simulink model "PhaseShiftedCarriers"  (R2023b)
settings: Solver=FixedStepAuto  StartTime=0.0  StopTime=4/ffund  FixedStep=1e-6  RelTol=1e-3
InitFcn:
  | fsw=50e3;
  | 
  | ma=0.9;
  | 
  | ffund=100;
  | 
  | phi_pf=acos(0.9);
  | % 15*pi/180;
  | 
  | sym= pi/6;
libraries: spsRMSLib x5, dspstat3 x2, simulink x1
settings Model: Creator=enesa  LastModifiedBy=enesa

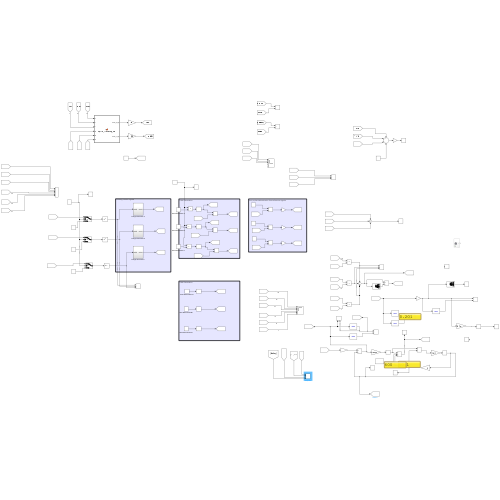
[thumbnail: Simulink's stored preview of the top-level diagram]
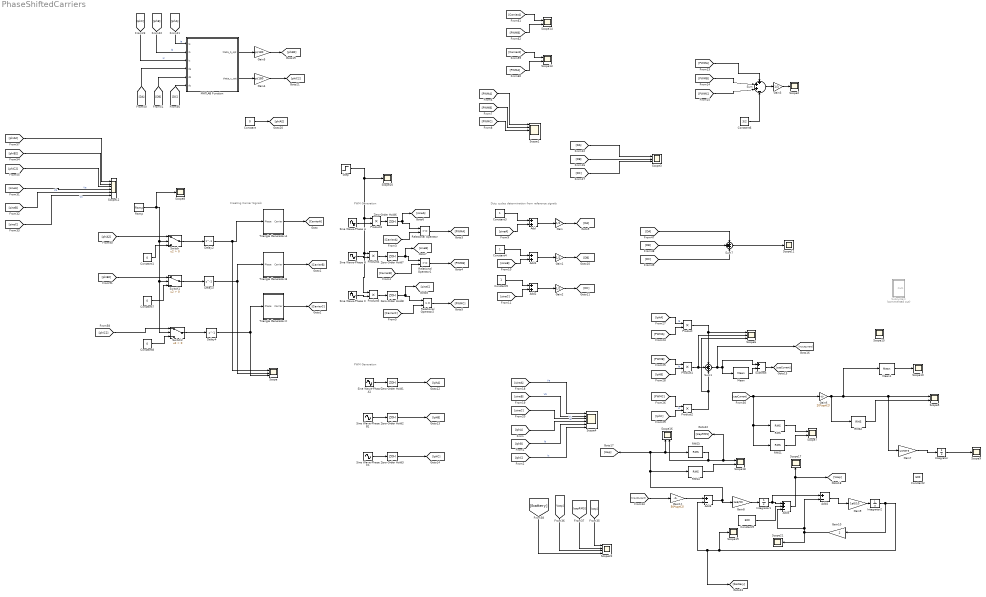
== system PhaseShiftedCarriers ==
  note: Duty cycles determination from reference signals
  note: PWM Generation
  note: Creating Carrier Signals
  note: PWM Generation
  Add : Sum
  Add1 : Sum
  Add2 : Sum
  Add3 : Sum  Inputs=+-
  Add4 : Sum  Inputs=+-
  Add5 : Sum  Inputs=++-
  Constant{,1,7..8} (4 alike) : Constant  Value=0
  Constant2 : Constant  Value=600
  Constant3 : Constant
  Constant4 : Constant
  Constant5 : Constant
  Constant6 : Constant  Value=3/2
  Constant9 : Constant  Value=600
  Delay2 : Delay  DelayLength=1  SampleTime=1/fsw
  Delay3 : Delay  DelayLength=1  SampleTime=1/fsw
  Delay4 : Delay  DelayLength=1  SampleTime=1/fsw
  Gain : Gain  Gain=1/2
  Gain1 : Gain  Gain=1/2
  Gain10 : Gain  Gain=2
  Gain11 : Gain  Gain=50*sqrt(2)
  Gain2 : Gain  Gain=1/2
  Gain3 : Gain  Gain=1/3
  Gain4 : Gain  Gain=pi/180
  Gain5 : Gain  Gain=pi/180
  Gain6 : Gain  Gain=20*sqrt(2)
  Gain7 : Gain  Gain=1/470e-6
  Gain8 : Gain  Gain=1e6/50
  Gain9 : Gain  Gain=1e6/10
  Integrator : Integrator
  Integrator1 : Integrator
  Integrator2 : Integrator
  MATLAB Function : MATLAB Function  TreatAsAtomicUnit=on
  Mean : dspstat3/Mean  run=on  InputProcessing=Columns as channels (frame based)  reset_popup=None  directionMode=Each column  dimension=1  roiEnable=off  roiType=Rectangles  roiPortion=Entire ROI  roiOutput=Individual statistics for each ROI  roiFlag=off  roundingMode=Floor  overflowMode=off  outputDataTypeStr=Inherit: Same as accumulator  outputMin=[]  outputMax=[]  outputLastDataTypeStr=Inherit: Same as accumulator
  Mean1 : dspstat3/Mean  run=on  reset_popup=None  directionMode=Each column  dimension=1  roiEnable=off  roiType=Rectangles  roiPortion=Entire ROI  roiOutput=Individual statistics for each ROI  roiFlag=off  roundingMode=Floor  overflowMode=off  outputDataTypeStr=Inherit: Same as accumulator  outputMin=[]  outputMax=[]  outputLastDataTypeStr=Inherit: Same as accumulator
  Product{,1..5} (6 alike) : Product
  RMS : spsRMSLib/RMS  TrueRMS=on  Freq=fsw  RMSInit=0  Ts=0
  RMS1 : spsRMSLib/RMS  TrueRMS=on  Freq=ffund  RMSInit=0  Ts=0
  RMS2 : spsRMSLib/RMS  TrueRMS=on  Freq=fsw  RMSInit=0  Ts=0
  RMS3 : spsRMSLib/RMS  TrueRMS=on  Freq=fsw  RMSInit=0  Ts=0
  RMS4 : spsRMSLib/RMS  TrueRMS=on  Freq=ffund  RMSInit=0  Ts=0
  Ramp : simulink/Sources/Ramp  slope=ffund/2  start=0  InitialOutput=-1
  Relational Operator : RelationalOperator  OutDataTypeStr=boolean  RndMeth=Simplest  InputSameDT=off
  Relational Operator1 : RelationalOperator  OutDataTypeStr=boolean  RndMeth=Simplest  InputSameDT=off
  Relational Operator2 : RelationalOperator  OutDataTypeStr=boolean  RndMeth=Simplest  InputSameDT=off
  Scope : Scope  NumInputPorts=3
  Scope1 : Scope  NumInputPorts=6
  Scope{2,8..11,15,17,19..21} (10 alike) : Scope
  Scope12 : Scope  NumInputPorts=6
  Scope{5,7,13..14,16,18} (6 alike) : Scope  NumInputPorts=2
  Scope22 : Scope  NumInputPorts=4
  Scope3 : Scope  NumInputPorts=3
  Scope4 : Scope  NumInputPorts=6
  Scope6 : Scope  NumInputPorts=3
  Sine Wave-Phase A : Sin  Amplitude=ma  Frequency=2*pi*ffund  SampleTime=0
  Sine Wave-Phase A1 : Sin  Amplitude=ma  Frequency=2*pi*ffund  Phase=0-phi_pf  SampleTime=0
  Sine Wave-Phase B : Sin  Amplitude=ma  Frequency=2*pi*ffund  Phase=2*pi/3  SampleTime=0
  Sine Wave-Phase B1 : Sin  Amplitude=ma  Frequency=2*pi*ffund  Phase=2*pi/3-phi_pf  SampleTime=0
  Sine Wave-Phase C : Sin  Amplitude=ma  Frequency=2*pi*ffund  Phase=-2*pi/3  SampleTime=0
  Sine Wave-Phase C1 : Sin  Amplitude=ma  Frequency=2*pi*ffund  Phase=-2*pi/3-phi_pf  SampleTime=0
  Step : Step  Time=8/ffund  Before=0.6/0.9  SampleTime=0
  Subsystem : Subsystem  Commented=on
  Subtract : Sum  Inputs=+-
  Sum : Sum  Inputs=+++-
  Sum1 : Sum  Inputs=+++
  Sum7 : Sum  Inputs=+++
  Switch : Switch  Criteria=u2 > Threshold  SaturateOnIntegerOverflow=off  InputSameDT=off
  Switch1 : Switch  Criteria=u2 > Threshold  SaturateOnIntegerOverflow=off  InputSameDT=off
  Switch2 : Switch  Criteria=u2 > Threshold  SaturateOnIntegerOverflow=off  InputSameDT=off
  Triangle Generator-A : Subsystem
  Triangle Generator-B : Subsystem
  Triangle Generator-C : Subsystem
  Zero-Order Hold{1..3,6..8} (6 alike) : ZeroOrderHold  SampleTime=5/fsw
  wires:
  [PWMA] -> Scope1/1
  [PWMB] -> Scope1/2
  [PWMC] -> Scope1/3
  [PWMA] -> Sum/1
  [PWMB] -> Sum/2
  [PWMC] -> Sum/3
  Sum/1 -> Gain3/1
  Gain3/1 -> Scope2/1
  Constant6/1 -> Sum/4
  [DA] -> Scope3/1
  [DB] -> Scope3/2
  [DC] -> Scope3/3
  Triangle Generator-C/1(Carrier) -> [CarrierC]
  Triangle Generator-B/1(Carrier) -> [CarrierB]
  Triangle Generator-A/1(Carrier) -> [CarrierA]
  [CarrierB] -> Relational Operator1/2
  Relational Operator1/1 -> [PWMB]
  Relational Operator/1 -> [PWMA]
  Relational Operator2/1 -> [PWMC]
  [CarrierC] -> Relational Operator2/2
  [CarrierA] -> Relational Operator/2
  [sineC] -> Add2/2
  Constant4/1 -> Add1/1
  Constant3/1 -> Add/1
  Add2/1 -> Gain2/1
  Gain/1 -> [DA]
  Gain2/1 -> [DC]
  Add1/1 -> Gain1/1
  [sineB] -> Add1/2
  Constant5/1 -> Add2/1
  [sineA] -> Add/2
  Gain1/1 -> [DB]
  Add/1 -> Gain/1
  [DA] -> Sum7/1
  [DC] -> Sum7/3
  [DB] -> Sum7/2
  Sum7/1 -> Scope11/1
  [phiB2] -> Scope12/2
  [phiC2] -> Scope12/3
  [phiA2] -> Scope12/1
  [CarrierA] -> Scope13/1
  [PWMA] -> Scope13/2
  [CarrierA] -> Scope14/1
  [PWMB] -> Scope14/2
  Gain4/1 -> [phiC2]
  Constant/1 -> [phiA2]
  Zero-Order Hold6/1 -> Relational Operator/1, [sineA]
  Zero-Order Hold7/1 -> [sineB], Relational Operator1/1
  Zero-Order Hold8/1 -> Relational Operator2/1, [sineC]
  Delay2/1 -> Scope/1, Triangle Generator-A/1(Phase)
  Delay3/1 -> Triangle Generator-B/1(Phase), Scope/2
  Delay4/1 -> Triangle Generator-C/1(Phase), Scope/3
  Zero-Order Hold1/1 -> [IphA]
  Zero-Order Hold2/1 -> [IphB]
  Sine Wave-Phase C1/1 -> Zero-Order Hold3/1
  Sine Wave-Phase B1/1 -> Zero-Order Hold2/1
  Zero-Order Hold3/1 -> [IphC]
  Sine Wave-Phase A1/1 -> Zero-Order Hold1/1
  [sineA] -> Scope4/1  "Va"
  [sineB] -> Scope4/2  "Vb"
  [sineC] -> Scope4/3  "Vc"
  [IphA] -> Scope4/4  "Ia"
  [IphB] -> Scope4/5  "Ib"
  [IphC] -> Scope4/6  "Ic"
  [DA] -> MATLAB Function/4(da)
  [DB] -> MATLAB Function/5(db)
  [DC] -> MATLAB Function/6(dc)
  [IphA] -> MATLAB Function/1(ia)  "Ia"
  [IphB] -> MATLAB Function/2(ib)  "Ib"
  [IphC] -> MATLAB Function/3(ic)  "Ic"
  MATLAB Function/1(theta_b_opt) -> Gain5/1
  MATLAB Function/2(theta_c_opt) -> Gain4/1
  Gain5/1 -> [phiB2]
  [IphA] -> Product/1  "Ia"
  [PWMA] -> Product/2
  [PWMB] -> Product1/1
  [IphB] -> Product1/2  "Ib"
  [PWMC] -> Product2/1
  [IphC] -> Product2/2  "Ic"
  Product/1 -> Sum1/1, Scope6/1
  Product1/1 -> Scope6/2, Sum1/2
  Product2/1 -> Scope6/3, Sum1/3
  [capCurrent] -> RMS1/1, RMS/1, Gain6/1
  Switch/1 -> Delay2/1
  [phiA2] -> Switch/1
  Constant1/1 -> Switch/3
  Ramp/1 -> Scope8/1, Switch2/2, Switch1/2, Switch/2
  Switch1/1 -> Delay3/1
  Constant7/1 -> Switch1/3
  [phiB2] -> Switch1/1
  Switch2/1 -> Delay4/1
  [phiC2] -> Switch2/1
  Constant8/1 -> Switch2/3
  RMS/1 -> Scope7/1
  [sineA] -> Scope12/4  "Va"
  [sineB] -> Scope12/5  "Vb"
  [sineC] -> Scope12/6  "Vc"
  RMS1/1 -> Scope7/2
  Sum1/1 -> [InputCurrent], Mean/1, Subtract/1
  Mean/1 -> Subtract/2
  Subtract/1 -> [capCurrent]
  Gain6/1 -> RMS2/1, Mean1/1, Gain7/1, Scope5/1
  RMS2/1 -> Scope5/2
  Gain7/1 -> Integrator/1
  Integrator/1 -> Scope9/1
  Mean1/1 -> Scope10/1
  [InputCurrent] -> Gain11/1
  Gain8/1 -> Integrator1/1
  Add4/1 -> Gain9/1
  Gain9/1 -> Integrator2/1
  Integrator2/1 -> Scope19/1, [Ibattery], Add3/2, Gain10/1
  Gain10/1 -> Add5/3, Add4/2, Scope21/1
  Integrator1/1 -> Add4/1, Add5/1
  Add5/1 -> Scope17/1, [Vcap]
  Gain11/1 -> Add3/1
  RMS4/1 -> Scope18/2
  Add3/1 -> Gain8/1, RMS3/1, Scope16/1, [Icap], RMS4/1
  RMS3/1 -> Scope16/2, [IcapRMS], Scope18/1
  Product3/1 -> Zero-Order Hold6/1
  Sine Wave-Phase A/1 -> Product3/2
  Step/1 -> Scope20/1, Product3/1, Product5/1, Product4/1
  Product4/1 -> Zero-Order Hold7/1
  Sine Wave-Phase B/1 -> Product4/2
  Product5/1 -> Zero-Order Hold8/1
  Sine Wave-Phase C/1 -> Product5/2
  Constant9/1 -> Add5/2
  [Icap] -> Scope22/1
  [Vcap] -> Scope22/3
  [IcapRMS] -> Scope22/2
  [Ibattery] -> Scope22/4

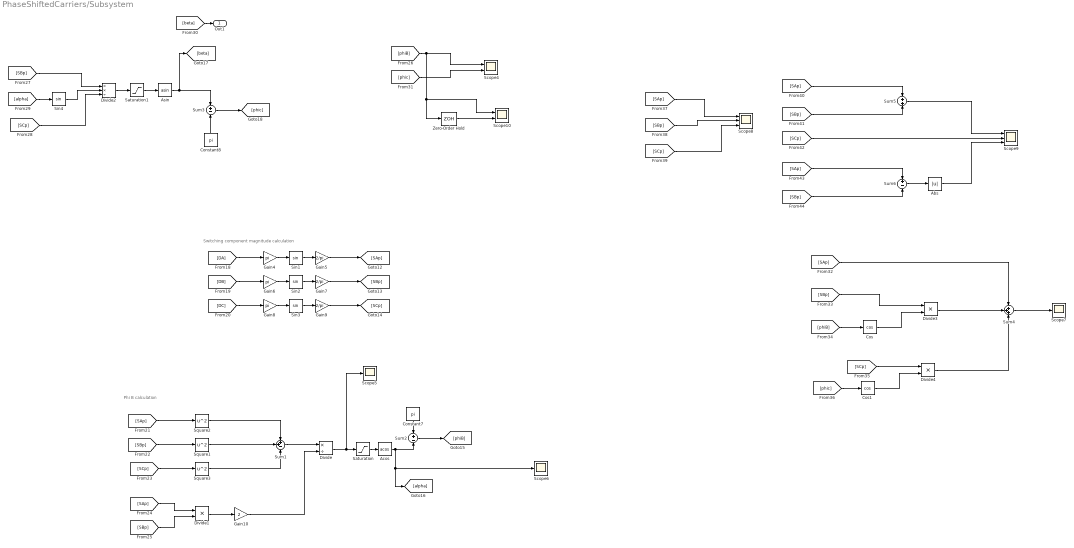
== system PhaseShiftedCarriers/Subsystem ==
  note: Phi B calculation
  note: Switching component magnitude calculation
  Abs : Abs  SaturateOnIntegerOverflow=off
  Acos : Trigonometry  Operator=acos
  Asin : Trigonometry  Operator=asin
  Constant7 : Constant  Value=pi
  Constant8 : Constant  Value=pi
  Cos : Trigonometry  Operator=cos
  Cos1 : Trigonometry  Operator=cos
  Divide : Product  Inputs=*/
  Divide1 : Product  Inputs=**
  Divide2 : Product  Inputs=**/
  Divide3 : Product  Inputs=**
  Divide4 : Product  Inputs=**
  Gain10 : Gain  Gain=2
  Gain4 : Gain  Gain=pi
  Gain5 : Gain  Gain=2/pi
  Gain6 : Gain  Gain=pi
  Gain7 : Gain  Gain=2/pi
  Gain8 : Gain  Gain=pi
  Gain9 : Gain  Gain=2/pi
  Saturation : Saturate  UpperLimit=1  LowerLimit=-1
  Saturation1 : Saturate  UpperLimit=1  LowerLimit=-1
  Scope10 : Scope  NumInputPorts=2
  Scope4 : Scope  NumInputPorts=2
  Scope5 : Scope
  Scope6 : Scope
  Scope7 : Scope
  Scope8 : Scope  NumInputPorts=3
  Scope9 : Scope  NumInputPorts=3
  Sin{1..4} (4 alike) : Trigonometry
  Square1 : Math  Operator=square
  Square2 : Math  Operator=square
  Square3 : Math  Operator=square
  Sum1 : Sum  Inputs=++-
  Sum2 : Sum  Inputs=+-
  Sum3 : Sum  Inputs=+-
  Sum4 : Sum  Inputs=+++
  Sum5 : Sum
  Sum6 : Sum  Inputs=+-
  Zero-Order Hold : ZeroOrderHold  SampleTime=1/fsw
  Out1 : Outport
  wires:
  Gain7/1 -> [SBp]
  Gain4/1 -> Sin1/1
  [SBp] -> Divide1/2
  Gain9/1 -> [SCp]
  Acos/1 -> Sum2/2, Scope6/1, [alpha]
  [beta] -> Out1/1
  Divide1/1 -> Gain10/1
  Asin/1 -> Sum3/1, [beta]
  Sin4/1 -> Divide2/2
  Gain6/1 -> Sin2/1
  Sin2/1 -> Gain7/1
  [DA] -> Gain4/1
  Gain10/1 -> Divide/2
  Gain5/1 -> [SAp]
  Sum1/1 -> Divide/1
  Square3/1 -> Sum1/3
  Square2/1 -> Sum1/1
  [SAp] -> Divide1/1
  [SBp] -> Square1/1
  Sum2/1 -> [phiB]
  [alpha] -> Sin4/1
  [SBp] -> Divide2/1
  [SCp] -> Divide2/3
  [DC] -> Gain8/1
  [SAp] -> Square2/1
  [phiB] -> Scope10/1, Zero-Order Hold/1, Scope4/1
  Sin1/1 -> Gain5/1
  Divide/1 -> Scope5/1, Saturation/1
  Constant8/1 -> Sum3/2
  Square1/1 -> Sum1/2
  [phic] -> Scope4/2
  Sin3/1 -> Gain9/1
  Saturation/1 -> Acos/1
  Saturation1/1 -> Asin/1
  [DB] -> Gain6/1
  Gain8/1 -> Sin3/1
  Divide2/1 -> Saturation1/1
  Zero-Order Hold/1 -> Scope10/2
  [SCp] -> Square3/1
  Sum3/1 -> [phic]
  Constant7/1 -> Sum2/1
  Cos1/1 -> Divide4/2
  [SBp] -> Scope8/2
  Abs/1 -> Scope9/3
  [SCp] -> Scope9/2
  [SAp] -> Scope8/1
  Sum5/1 -> Scope9/1
  [SBp] -> Sum6/2
  [SAp] -> Sum6/1
  Cos/1 -> Divide3/2
  [SBp] -> Sum5/2
  [SAp] -> Sum4/1
  [SCp] -> Scope8/3
  Sum4/1 -> Scope7/1
  Sum6/1 -> Abs/1
  [SAp] -> Sum5/1
  [SBp] -> Divide3/1
  Divide4/1 -> Sum4/3
  [phiB] -> Cos/1
  Divide3/1 -> Sum4/2
  [SCp] -> Divide4/1
  [phic] -> Cos1/1

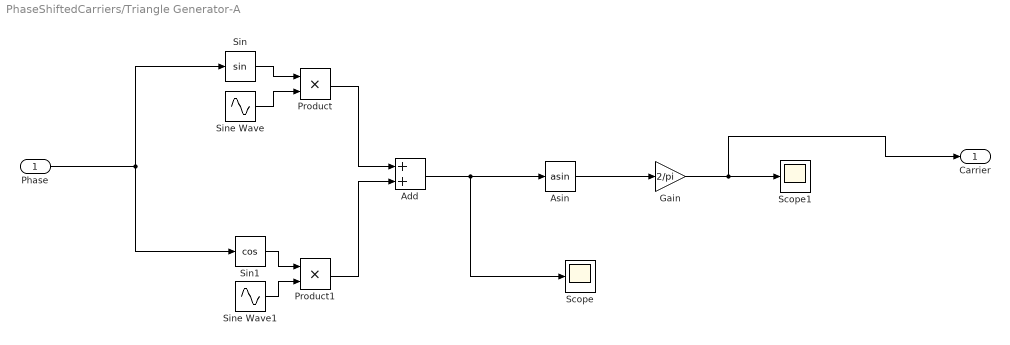
== system PhaseShiftedCarriers/Triangle Generator-A ==
  Phase : Inport
  Add : Sum
  Asin : Trigonometry  Operator=asin
  Gain : Gain  Gain=2/pi
  Product : Product
  Product1 : Product
  Scope : Scope
  Scope1 : Scope
  Sin : Trigonometry
  Sin1 : Trigonometry  Operator=cos
  Sine Wave : Sin  Frequency=2*pi*fsw  SampleTime=0
  Sine Wave1 : Sin  Frequency=2*pi*fsw  Phase=-pi/2  SampleTime=0
  Carrier : Outport
  wires:
  Sin/1 -> Product/1
  Sine Wave/1 -> Product/2
  Phase/1 -> Sin/1, Sin1/1
  Product/1 -> Add/1
  Asin/1 -> Gain/1
  Gain/1 -> Carrier/1, Scope1/1
  Sine Wave1/1 -> Product1/2
  Product1/1 -> Add/2
  Add/1 -> Asin/1, Scope/1
  Sin1/1 -> Product1/1

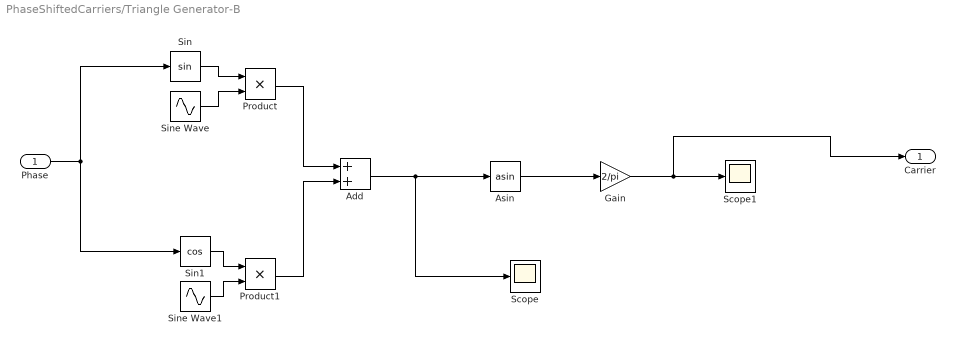
== system PhaseShiftedCarriers/Triangle Generator-B ==
  Phase : Inport
  Add : Sum
  Asin : Trigonometry  Operator=asin
  Gain : Gain  Gain=2/pi
  Product : Product
  Product1 : Product
  Scope : Scope
  Scope1 : Scope
  Sin : Trigonometry
  Sin1 : Trigonometry  Operator=cos
  Sine Wave : Sin  Frequency=2*pi*fsw  SampleTime=0
  Sine Wave1 : Sin  Frequency=2*pi*fsw  Phase=-pi/2  SampleTime=0
  Carrier : Outport
  wires:
  Sin/1 -> Product/1
  Sine Wave/1 -> Product/2
  Phase/1 -> Sin1/1, Sin/1
  Product/1 -> Add/1
  Asin/1 -> Gain/1
  Gain/1 -> Carrier/1, Scope1/1
  Sine Wave1/1 -> Product1/2
  Product1/1 -> Add/2
  Add/1 -> Asin/1, Scope/1
  Sin1/1 -> Product1/1

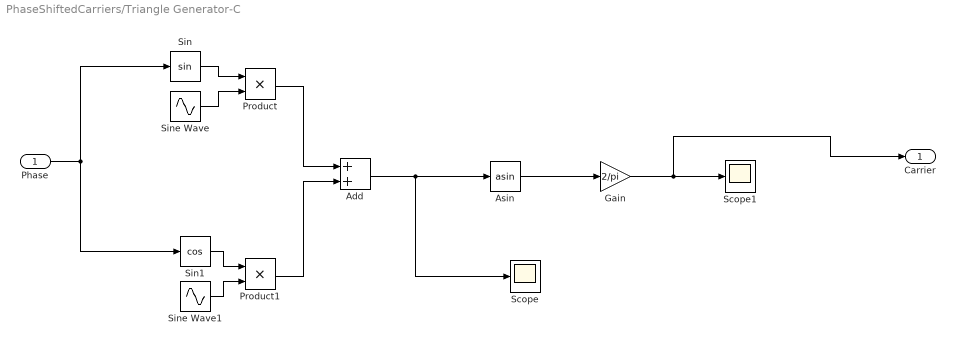
== system PhaseShiftedCarriers/Triangle Generator-C ==
  Phase : Inport
  Add : Sum
  Asin : Trigonometry  Operator=asin
  Gain : Gain  Gain=2/pi
  Product : Product
  Product1 : Product
  Scope : Scope
  Scope1 : Scope
  Sin : Trigonometry
  Sin1 : Trigonometry  Operator=cos
  Sine Wave : Sin  Frequency=2*pi*fsw  SampleTime=0
  Sine Wave1 : Sin  Frequency=2*pi*fsw  Phase=-pi/2  SampleTime=0
  Carrier : Outport
  wires:
  Sin/1 -> Product/1
  Sine Wave/1 -> Product/2
  Phase/1 -> Sin1/1, Sin/1
  Product/1 -> Add/1
  Asin/1 -> Gain/1
  Gain/1 -> Carrier/1, Scope1/1
  Sine Wave1/1 -> Product1/2
  Product1/1 -> Add/2
  Add/1 -> Asin/1, Scope/1
  Sin1/1 -> Product1/1

== matlab function PhaseShiftedCarriers/MATLAB Function ==
  data: ia input; ib input; ic input; theta_b_opt output; da input; db input; theta_c_opt output; dc input
function [theta_b_opt, theta_c_opt] = optimize_interleaving_rms(ia, ib, ic, da, db, dc)

    % Simulation parameters
    fsw = 10e3;
    Ts = 1/fsw;
    N = 1000;
    t = linspace(0, Ts, N);

    % Reference triangular carrier for phase A
    carrier = sawtooth(2*pi*fsw*t, 0.5);  % symmetric triangle [-1,1]

    % Initialize results
    min_rms = Inf;
    theta_b_opt = 0;
    theta_c_opt = 0;

    % Search over all combinations of θ_b and θ_c
    for theta_b = 0:5:360
    for theta_c = 0:5:360

            % Convert angle to carrier time shift
            shift_b = mod(theta_b / 360, 1) * Ts;
            shift_c = mod(theta_c / 360, 1) * Ts;

            % Create phase-shifted carriers
            carrier_b = sawtooth(2*pi*fsw*(t - shift_b), 0.5);
            carrier_c = sawtooth(2*pi*fsw*(t - shift_c), 0.5);

            % Switching functions
            sa = 2*da-1 >= carrier;
            sb = 2*db-1 >= carrier_b;
            sc = 2*dc-1 >= carrier_c;

            % DC-link current: sum of absolute leg currents
            idc = sa.* ia + sb.* ib +sc .* ic-mean(sa.* ia + sb.* ib +sc .* ic);
            rms_val = sqrt(mean(idc.^2));

            if rms_val < min_rms
                min_rms = rms_val;
                theta_b_opt = theta_b;
                theta_c_opt = theta_c;
            end
        end
    end
end
